simulink subsystem "BEV_MockModel_refsub"  (R2026a)
settings: Solver=VariableStepAuto  StopTime=600
undefined symbols (not defined in the file or in its folder): bevControl
settings Model: Creator=isaacito  LastModifiedBy=isaacito

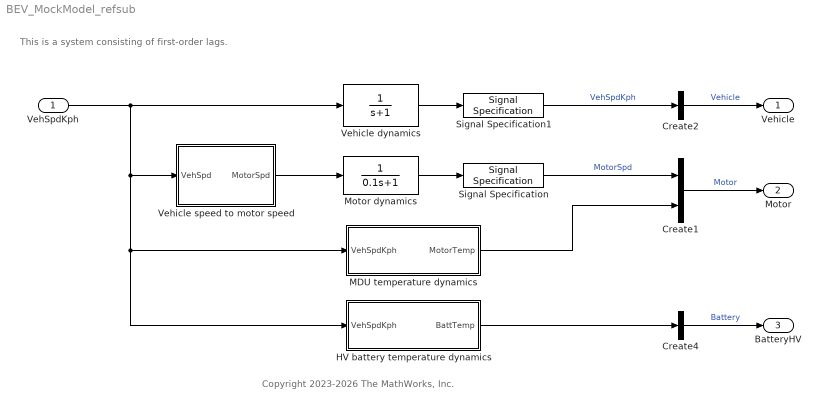
== system BEV_MockModel_refsub ==
  note: This is a system consisting of first-order lags.
  note: Copyright 2023-2026 The MathWorks, Inc.
  VehSpdKph : Inport
  Create1 : BusCreator  Inputs=2
  Create2 : BusCreator  Inputs=1
  Create4 : BusCreator  Inputs=1
  HV battery temperature dynamics : Subsystem
  MDU temperature dynamics : Subsystem
  Motor dynamics : TransferFcn  Denominator=[0.1 1]
  Signal Specification : SignalSpecification  Unit=rpm
  Signal Specification1 : SignalSpecification  Unit=km/h
  Vehicle dynamics : TransferFcn  Denominator=[1 1]
  Vehicle speed to motor speed : Subsystem
  Vehicle : Outport
  Motor : Outport  Port=2
  BatteryHV : Outport  Port=3
  wires:
  Vehicle speed to motor speed/1(MotorSpd) -> Motor dynamics/1
  Create2/1 -> Vehicle/1  "Vehicle"
  Create1/1 -> Motor/1  "Motor"
  Vehicle dynamics/1 -> Signal Specification1/1
  VehSpdKph/1 -> Vehicle speed to motor speed/1(VehSpd), MDU temperature dynamics/1(VehSpdKph), HV battery temperature dynamics/1(VehSpdKph), Vehicle dynamics/1
  Create4/1 -> BatteryHV/1  "Battery"
  HV battery temperature dynamics/1(BattTemp) -> Create4/1
  MDU temperature dynamics/1(MotorTemp) -> Create1/2
  Signal Specification1/1 -> Create2/1  "VehSpdKph"
  Signal Specification/1 -> Create1/1  "MotorSpd"
  Motor dynamics/1 -> Signal Specification/1

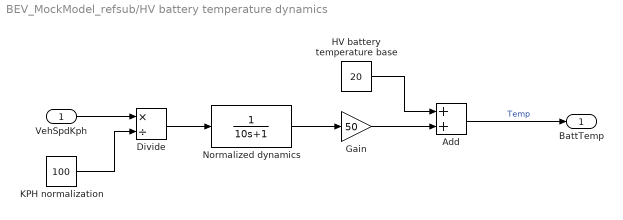
== system BEV_MockModel_refsub/HV battery temperature dynamics ==
  VehSpdKph : Inport  Unit=km/hr
  Add : Sum
  Divide : Product  Inputs=*/
  Gain : Gain  Gain=50
  HV battery temperature base : Constant  Value=20
  KPH normalization : Constant  Value=100
  Normalized dynamics : TransferFcn  Denominator=[10 1]
  BattTemp : Outport  Unit=degC
  wires:
  VehSpdKph/1 -> Divide/1
  Normalized dynamics/1 -> Gain/1
  Divide/1 -> Normalized dynamics/1
  HV battery temperature base/1 -> Add/1
  Gain/1 -> Add/2
  Add/1 -> BattTemp/1  "Temp"
  KPH normalization/1 -> Divide/2

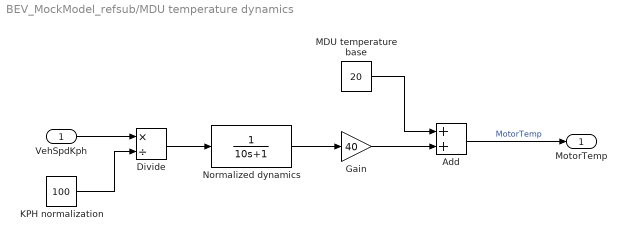
== system BEV_MockModel_refsub/MDU temperature dynamics ==
  VehSpdKph : Inport  Unit=km/hr
  Add : Sum
  Divide : Product  Inputs=*/
  Gain : Gain  Gain=40
  KPH normalization : Constant  Value=100
  MDU temperature base : Constant  Value=20
  Normalized dynamics : TransferFcn  Denominator=[10 1]
  MotorTemp : Outport  Unit=degC
  wires:
  VehSpdKph/1 -> Divide/1
  Normalized dynamics/1 -> Gain/1
  Divide/1 -> Normalized dynamics/1
  MDU temperature base/1 -> Add/1
  Gain/1 -> Add/2
  Add/1 -> MotorTemp/1  "MotorTemp"
  KPH normalization/1 -> Divide/2

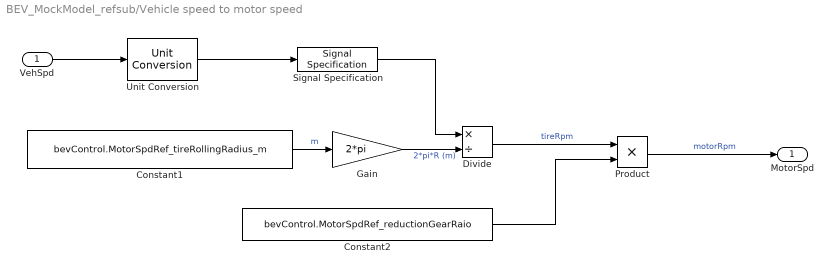
== system BEV_MockModel_refsub/Vehicle speed to motor speed ==
  VehSpd : Inport  Unit=km/hr
  Constant1 : Constant  Value=bevControl.MotorSpdRef_tireRollingRadius_m
  Constant2 : Constant  Value=bevControl.MotorSpdRef_reductionGearRaio
  Divide : Product  Inputs=*/
  Gain : Gain  Gain=2*pi
  Product : Product
  Signal Specification : SignalSpecification  Unit=m/min
  Unit Conversion : UnitConversion
  MotorSpd : Outport  Unit=rpm  VectorParamsAs1DForOutWhenUnconnected=off
  wires:
  VehSpd/1 -> Unit Conversion/1
  Unit Conversion/1 -> Signal Specification/1
  Signal Specification/1 -> Divide/1
  Gain/1 -> Divide/2  "2*pi*R (m)"
  Divide/1 -> Product/1  "tireRpm"
  Constant2/1 -> Product/2
  Product/1 -> MotorSpd/1  "motorRpm"
  Constant1/1 -> Gain/1  "m"
